simulink model "Roesssler_Try"  (R2024b)
settings: Solver=FixedStepAuto  StartTime=0.0  StopTime=100.0  FixedStep=0.01  RelTol=1e-3
settings Model: Creator=max  LastModifiedBy=max

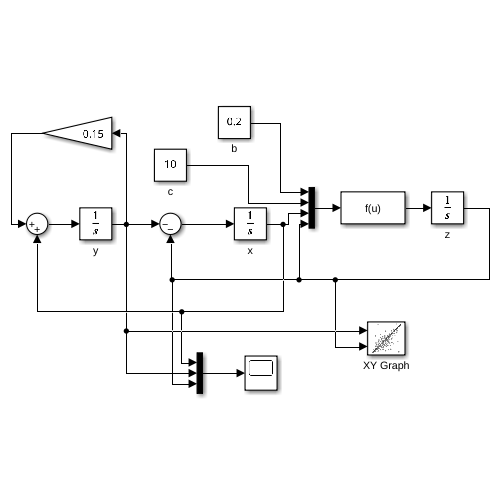
[thumbnail: Simulink's stored preview of the top-level diagram]
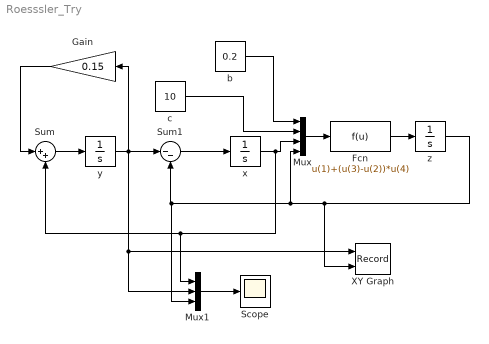
== system Roesssler_Try ==
  Fcn : Fcn  Expr=u(1)+(u(3)-u(2))*u(4)
  Gain : Gain  Gain=0.15
  Mux : Mux
  Mux1 : Mux  Inputs=3
  Scope : Scope
  Sum : Sum  Inputs=|++
  Sum1 : Sum  Inputs=|--
  XY Graph : Record  FileSettingsInternal="{\"entries\":[{\"content\":{\"excelSettings\":{\"content\":{},\"type\":\"Streamout.ExcelSettings\"}},\"type\":\"Streamout.FileSettingStorage\",\"uuid\":\"\"}],\"packageUris\":[\"http:\\/\\/schema.mathworks.com\\/mf0\\/streamout_blocks\\/R2020a\"],\"version\":\"1.0\"}"  Layout=[1 1]  SignalsInternal="{\"entries\":[{\"content\":{\"signals\":[{\"content\":{\"blockPath\":[],\"dimensions\":[1],\"domain\":\"\",\"lineColor\":\"#a2142f\",\"plots\":[ 1 ],\"port\":1,\"sid\":[\"\"],\"signalID\":1,\"signalName\":\"y\"},\"type\":\"RecordBlkView.Signal\",\"uuid\":\"\"},{\"content\":{\"blockPath\":[],\"dimensions\":[1],\"domain\":\"\",\"lineColor\":\"#139fff\",\"plots\":[ 1 ],\"port\":2,\"sid\":[\"\"],\"signalID\":2,\"signalName\":\"z\"},\"type\":\"RecordBlkView.Signal\",\"uuid\":\"\"}]},\"type\":\"RecordBlkView.InputSignals\",\"uuid\":\"\"}],\"packageUris\":[\"http:\\/\\/schema.mathworks.com\\/mf0\\/streamout_blocks\\/R2020a\"],\"version\":\"1.0\"}"  VisualizationBindings="{\"xyplotplugin\":{\"info\":[{\"series\":[{\"bindingParametersList\":[{\"parameter\":\"X-Axis\",\"signalID\":1,\"signalName\":\"y\"},{\"parameter\":\"Y-Axis\",\"signalID\":2,\"signalName\":\"z\"}],\"seriesID\":0}],\"subplotID\":1}]}}"  CompatibilityTag=XY
  b : Constant  Value=0.2
  c : Constant  Value=10
  x : Integrator
  y : Integrator
  z : Integrator
  wires:
  Sum/1 -> y/1
  Gain/1 -> Sum/1
  y/1 -> Mux1/2, XY Graph/1, Gain/1, Sum1/1
  Sum1/1 -> x/1
  c/1 -> Mux/2
  b/1 -> Mux/1
  Mux/1 -> Fcn/1
  Fcn/1 -> z/1
  z/1 -> XY Graph/2, Mux/4, Mux1/3, Sum1/2
  x/1 -> Mux/3, Mux1/1, Sum/2
  Mux1/1 -> Scope/1
